simulink model "Elec_Engg_10_03_01_motor"  (Simulink 6.1)
settings: Solver=ode45  StartTime=0.0  StopTime=100  RelTol=1e-3
values from neighbouring files (symbols this model uses):
  ambient = am    [Elec_Engg_10_03_01.m]    (also in Elec_Engg_10_03_011.m)
  slp = input('Enter slope:')    [Elec_Engg_10_03_01_simuliknk.m]
  temp_rpm = [15 16 17 18 19 20 21 22 23 24 25 26 ... (42 elements, 21x2)]    [var.mat]
libraries: simulink x3
settings Model: LastModifiedBy=vijay
settings DebuggingCC: SolverPrmCheckMsg=warning

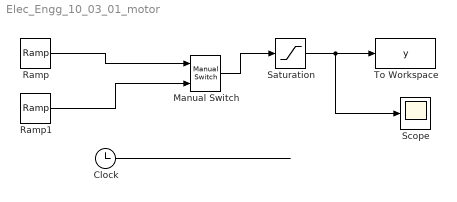
== system Elec_Engg_10_03_01_motor ==
  Clock : Clock
      settings: Decimation=10
  Manual Switch : simulink/Signal Routing/Manual Switch  sw=1  action=0
  Ramp : simulink/Sources/Ramp  slope=slp  start=0  X0=0
  Ramp1 : simulink/Sources/Ramp  slope=-slp  start=0  X0=0
  Saturation : Saturate  UpperLimit=temp_rpm(ambient-14,2)  LowerLimit=-temp_rpm(ambient-14,2)
  Scope : Scope
  To Workspace : ToWorkspace  VariableName=y  SampleTime=-1  SaveFormat=Structure
  wires:
  Ramp/1 -> Manual Switch/1
  Ramp1/1 -> Manual Switch/2
  Manual Switch/1 -> Saturation/1
  Saturation/1 -> To Workspace/1, Scope/1
  Clock/1 -> ?
